simulink subsystem "PurePursuitSubsystem"  (R2021b)
settings: Solver=VariableStepAuto  StartTime=0.0  StopTime=10.0  RelTol=1e-3
settings Model: Creator=ferna  LastModifiedBy=ferna

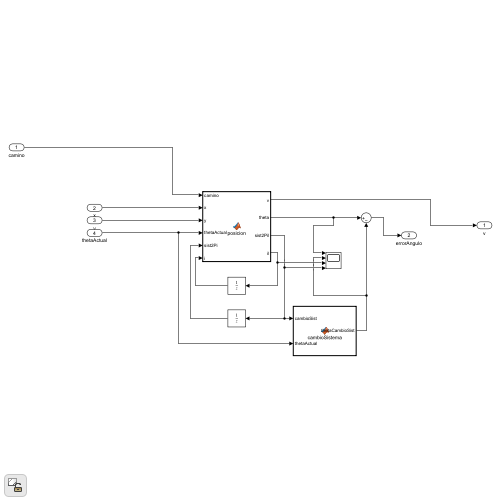
[thumbnail: Simulink's stored preview of the top-level diagram]
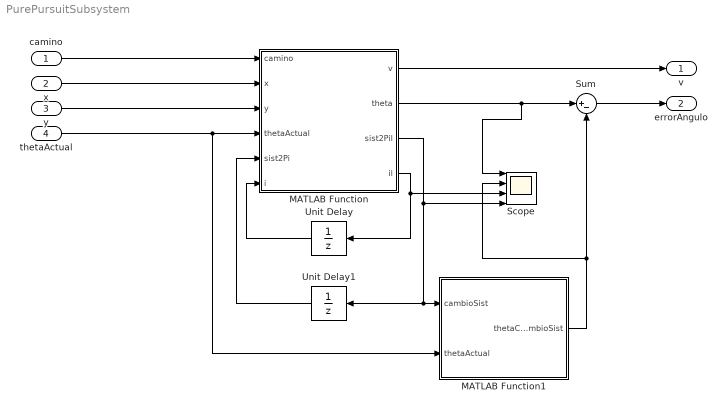
== system PurePursuitSubsystem ==
  camino : Inport
  x : Inport  Port=2
  y : Inport  Port=3
  thetaActual : Inport  Port=4
  MATLAB Function : MATLAB Function  TreatAsAtomicUnit=on
  MATLAB Function1 : MATLAB Function  TreatAsAtomicUnit=on
  Scope : Scope  NumInputPorts=4
  Sum : Sum  Inputs=|+-
  Unit Delay : UnitDelay  SampleTime=-1  HasFrameUpgradeWarning=on
  Unit Delay1 : UnitDelay  SampleTime=-1  HasFrameUpgradeWarning=on
  v : Outport
  errorAngulo : Outport  Port=2
  wires:
  MATLAB Function/2(theta) -> Sum/1, Scope/1
  thetaActual/1 -> MATLAB Function1/2(thetaActual), MATLAB Function/4(thetaActual)
  MATLAB Function/3(sist2Pil) -> Scope/4, MATLAB Function1/1(cambioSist), Unit Delay1/1
  y/1 -> MATLAB Function/3(y)
  MATLAB Function1/1(thetaCambioSist) -> Sum/2, Scope/2
  Unit Delay1/1 -> MATLAB Function/5(sist2Pi)
  MATLAB Function/1(v) -> v/1
  MATLAB Function/4(il) -> Scope/3, Unit Delay/1
  Unit Delay/1 -> MATLAB Function/6(i)
  camino/1 -> MATLAB Function/1(camino)
  Sum/1 -> errorAngulo/1
  x/1 -> MATLAB Function/2(x)

== matlab function PurePursuitSubsystem/MATLAB Function1 ==
  data: cambioSist input; thetaActual input; thetaCambioSist output
function thetaCambioSist = cambioSistema(cambioSist, thetaActual)

if cambioSist == 1 && thetaActual < 0
    thetaCambioSist = thetaActual + 2*pi;
else
    thetaCambioSist = thetaActual;
end

== matlab function PurePursuitSubsystem/MATLAB Function ==
  data: camino input; v output; x input; y input; thetaActual input; sist2Pi input; i input; theta output; sist2Pil output; il output
function [v, theta, sist2Pil, il] = posicion (camino, x, y, thetaActual, sist2Pi, i)

    % Inicializamos variables de salida
    
    L=0.20; % distancia de persecucion
    v=0.3; % velocidad del robot
    margen = 0.2; % margen para que la función atan2 no de problemas
    
    
    if length(camino) >= i % mientras haya camino

        if thetaActual < 0.05 && i == 0
            theta = 0.05;
        else
           
            if i == 0
                i = 1;
                theta = (atan2((camino(i,2) - y), ((camino(i,1)) - x)));
                if thetaActual > 0 && theta < 0
                        if (thetaActual - theta) > pi
                            sist2Pi = 1;
                        end
                else
                    sist2Pi = 0;
                end
        
                if thetaActual < 0 && theta > 0
                    if (theta - thetaActual) > pi
                        sist2Pi = 1;
                    end
                end
            end
        
            % Calculamos distancia al objetivo
        
            distancia=sqrt((camino(i,1) -x)^2 + (camino(i,2)-y)^2);
            
            
            while ((distancia < L) && (length(camino) > i)) % ya hemos llegado
                %thetaActual = theta;
                i=i+1; % actualizar el objetivo
                theta = (atan2((camino(i,2) - y), ((camino(i,1)) - x)));
                distancia = sqrt((camino (i,1) -x)^2 + (camino (i, 2) -y)^2);
                
                if thetaActual > 0 && theta < 0
                    if (thetaActual - theta) > pi
                        sist2Pi = 1;
                    end
                else
                    sist2Pi = 0;
                end
    
                if thetaActual < 0 && theta > 0
                    if (theta - thetaActual) > pi
                        sist2Pi = 1;
                    end
                end
            end
            
            %Calculo de la orientacion al punto i-esimo 
            theta = (atan2((camino(i,2) - y), ((camino(i,1)) - x)));
            if sist2Pi == 1 && thetaActual < 0 && theta < 0
                theta = 2*pi + theta;
            end
            
    
            if i > 1
                if distancia < margen
                v = 0.2;
                end
                distanciaAnterior = sqrt((camino(i-1,1) -x)^2 + (camino(i-1,2)-y)^2);
                if distanciaAnterior < margen
                    v = 0.2;
                end
            end
            
            if (distancia < (L/2)) && (length(camino) == i)
                i = i+1;
            end
         end
        

    else % si se ha llegado al final del camino

        theta = 0;
        v = 0;
    
    end
    il = i;
    sist2Pil = sist2Pi;

end
